simulink model "fftanalyzeri"  (R2012b)
settings: Solver=ode3  SolverMode=SingleTasking  StartTime=0.0  StopTime=20000  RelTol=1e-3
undefined symbols (not defined in the file or in its folder): pfb_coeff_gen_calc
undefined symbols (not defined in the file): fft_bin_flags_, magphmeanmem_, threshmem_
libraries: xbsIndex_r4 x9073, casper_library_misc x119, casper_library_flow_control x51, casper_library_delays x22, xps_library x10
(part 18 of 74)

== system fftanalyzeri/FIFO64_/FIFO32_0/FIFO16Cir_1/CounterArray2 ==
  chan : Inport
  inc : Inport  Port=2
  rst : Inport  Port=3
  chan2 : Inport  Port=4
  Mux : xbsIndex_r4/Mux  inputs=16  en=off  latency=0  precision=Full  arith_type=Unsigned  n_bits=16  bin_pt=14  quantization=Truncate  overflow=Wrap  dbl_ovrd=off  block_type=mux
  Mux1 : xbsIndex_r4/Mux  inputs=16  en=off  latency=0  precision=Full  arith_type=Unsigned  n_bits=16  bin_pt=14  quantization=Truncate  overflow=Wrap  dbl_ovrd=off  block_type=mux
  T1_4_{,1..15} (16 alike) : xbsIndex_r4/Counter  cnt_type=Free Running  cnt_to=Inf  operation=Up  start_count=0  cnt_by_val=1  arith_type=Unsigned  n_bits=8  bin_pt=0  load_pin=off  rst=on  en=on  explicit_period=on  period=1  dbl_ovrd=off  use_behavioral_HDL=off  implementation=Fabric  block_type=counter
  demux16_ : Subsystem
  Out1 : Outport
  Out2 : Outport  Port=2
  wires:
  chan/1 -> Mux/1, demux16_/1(Chan)
  inc/1 -> demux16_/2(din)
  rst/1 -> T1_4_9/1, T1_4_10/1, T1_4_11/1, T1_4_15/1, T1_4_8/1, T1_4_12/1, T1_4_14/1, T1_4_13/1, T1_4_7/1, T1_4_5/1, T1_4_1/1, T1_4_/1, T1_4_2/1, T1_4_3/1, T1_4_4/1, T1_4_6/1
  demux16_/1(Out1) -> T1_4_/2
  demux16_/2(Out2) -> T1_4_1/2
  demux16_/3(Out3) -> T1_4_2/2
  demux16_/4(Out4) -> T1_4_3/2
  demux16_/5(Out5) -> T1_4_4/2
  demux16_/6(Out6) -> T1_4_5/2
  demux16_/7(Out7) -> T1_4_6/2
  demux16_/8(Out8) -> T1_4_7/2
  demux16_/9(Out9) -> T1_4_9/2
  demux16_/10(Out10) -> T1_4_10/2
  demux16_/11(Out11) -> T1_4_11/2
  demux16_/12(Out12) -> T1_4_15/2
  demux16_/13(Out13) -> T1_4_8/2
  demux16_/14(Out14) -> T1_4_12/2
  demux16_/15(Out15) -> T1_4_13/2
  demux16_/16(Out16) -> T1_4_14/2
  T1_4_/1 -> Mux1/2, Mux/2
  T1_4_1/1 -> Mux1/3, Mux/3
  T1_4_2/1 -> Mux1/4, Mux/4
  T1_4_3/1 -> Mux1/5, Mux/5
  T1_4_4/1 -> Mux/6, Mux1/6
  T1_4_5/1 -> Mux1/7, Mux/7
  T1_4_6/1 -> Mux1/8, Mux/8
  T1_4_7/1 -> Mux1/9, Mux/9
  T1_4_9/1 -> Mux1/10, Mux/10
  T1_4_10/1 -> Mux1/11, Mux/11
  T1_4_11/1 -> Mux1/12, Mux/12
  T1_4_15/1 -> Mux1/13, Mux/13
  T1_4_8/1 -> Mux1/14, Mux/14
  T1_4_12/1 -> Mux1/15, Mux/15
  T1_4_13/1 -> Mux1/16, Mux/16
  T1_4_14/1 -> Mux/17, Mux1/17
  Mux/1 -> Out1/1
  chan2/1 -> Mux1/1
  Mux1/1 -> Out2/1

== system fftanalyzeri/FIFO64_/FIFO32_0/FIFO16Cir_2/CounterArray1 ==
  chan : Inport
  inc : Inport  Port=2
  rst : Inport  Port=3
  Mux : xbsIndex_r4/Mux  inputs=16  en=off  latency=0  precision=Full  arith_type=Unsigned  n_bits=16  bin_pt=14  quantization=Truncate  overflow=Wrap  dbl_ovrd=off  block_type=mux
  T1_4_{,1..15} (16 alike) : xbsIndex_r4/Counter  cnt_type=Free Running  cnt_to=Inf  operation=Up  start_count=0  cnt_by_val=1  arith_type=Unsigned  n_bits=8  bin_pt=0  load_pin=off  rst=on  en=on  explicit_period=on  period=1  dbl_ovrd=off  use_behavioral_HDL=off  implementation=Fabric  block_type=counter
  demux16_ : Subsystem
  Out1 : Outport
  wires:
  chan/1 -> Mux/1, demux16_/1(Chan)
  inc/1 -> demux16_/2(din)
  rst/1 -> T1_4_9/1, T1_4_10/1, T1_4_11/1, T1_4_12/1, T1_4_8/1, T1_4_13/1, T1_4_15/1, T1_4_14/1, T1_4_7/1, T1_4_6/1, T1_4_5/1, T1_4_4/1, T1_4_3/1, T1_4_2/1, T1_4_1/1, T1_4_/1
  demux16_/1(Out1) -> T1_4_/2
  demux16_/2(Out2) -> T1_4_1/2
  demux16_/3(Out3) -> T1_4_2/2
  demux16_/4(Out4) -> T1_4_3/2
  demux16_/5(Out5) -> T1_4_4/2
  demux16_/6(Out6) -> T1_4_5/2
  demux16_/7(Out7) -> T1_4_6/2
  demux16_/8(Out8) -> T1_4_7/2
  demux16_/9(Out9) -> T1_4_9/2
  demux16_/10(Out10) -> T1_4_10/2
  demux16_/11(Out11) -> T1_4_11/2
  demux16_/12(Out12) -> T1_4_12/2
  demux16_/13(Out13) -> T1_4_8/2
  demux16_/14(Out14) -> T1_4_13/2
  demux16_/15(Out15) -> T1_4_14/2
  demux16_/16(Out16) -> T1_4_15/2
  T1_4_/1 -> Mux/2
  T1_4_1/1 -> Mux/3
  T1_4_2/1 -> Mux/4
  T1_4_3/1 -> Mux/5
  T1_4_4/1 -> Mux/6
  T1_4_5/1 -> Mux/7
  T1_4_6/1 -> Mux/8
  T1_4_7/1 -> Mux/9
  T1_4_9/1 -> Mux/10
  T1_4_10/1 -> Mux/11
  T1_4_11/1 -> Mux/12
  T1_4_12/1 -> Mux/13
  T1_4_8/1 -> Mux/14
  T1_4_13/1 -> Mux/15
  T1_4_14/1 -> Mux/16
  T1_4_15/1 -> Mux/17
  Mux/1 -> Out1/1

== system fftanalyzeri/FIFO64_/FIFO32_0/FIFO16Cir_2/CounterArray2 ==
  chan : Inport
  inc : Inport  Port=2
  rst : Inport  Port=3
  chan2 : Inport  Port=4
  Mux : xbsIndex_r4/Mux  inputs=16  en=off  latency=0  precision=Full  arith_type=Unsigned  n_bits=16  bin_pt=14  quantization=Truncate  overflow=Wrap  dbl_ovrd=off  block_type=mux
  Mux1 : xbsIndex_r4/Mux  inputs=16  en=off  latency=0  precision=Full  arith_type=Unsigned  n_bits=16  bin_pt=14  quantization=Truncate  overflow=Wrap  dbl_ovrd=off  block_type=mux
  T1_4_{,1..15} (16 alike) : xbsIndex_r4/Counter  cnt_type=Free Running  cnt_to=Inf  operation=Up  start_count=0  cnt_by_val=1  arith_type=Unsigned  n_bits=8  bin_pt=0  load_pin=off  rst=on  en=on  explicit_period=on  period=1  dbl_ovrd=off  use_behavioral_HDL=off  implementation=Fabric  block_type=counter
  demux16_ : Subsystem
  Out1 : Outport
  Out2 : Outport  Port=2
  wires:
  chan/1 -> Mux/1, demux16_/1(Chan)
  inc/1 -> demux16_/2(din)
  rst/1 -> T1_4_9/1, T1_4_10/1, T1_4_11/1, T1_4_15/1, T1_4_8/1, T1_4_12/1, T1_4_14/1, T1_4_13/1, T1_4_7/1, T1_4_5/1, T1_4_1/1, T1_4_/1, T1_4_2/1, T1_4_3/1, T1_4_4/1, T1_4_6/1
  demux16_/1(Out1) -> T1_4_/2
  demux16_/2(Out2) -> T1_4_1/2
  demux16_/3(Out3) -> T1_4_2/2
  demux16_/4(Out4) -> T1_4_3/2
  demux16_/5(Out5) -> T1_4_4/2
  demux16_/6(Out6) -> T1_4_5/2
  demux16_/7(Out7) -> T1_4_6/2
  demux16_/8(Out8) -> T1_4_7/2
  demux16_/9(Out9) -> T1_4_9/2
  demux16_/10(Out10) -> T1_4_10/2
  demux16_/11(Out11) -> T1_4_11/2
  demux16_/12(Out12) -> T1_4_15/2
  demux16_/13(Out13) -> T1_4_8/2
  demux16_/14(Out14) -> T1_4_12/2
  demux16_/15(Out15) -> T1_4_13/2
  demux16_/16(Out16) -> T1_4_14/2
  T1_4_/1 -> Mux1/2, Mux/2
  T1_4_1/1 -> Mux1/3, Mux/3
  T1_4_2/1 -> Mux1/4, Mux/4
  T1_4_3/1 -> Mux1/5, Mux/5
  T1_4_4/1 -> Mux/6, Mux1/6
  T1_4_5/1 -> Mux1/7, Mux/7
  T1_4_6/1 -> Mux1/8, Mux/8
  T1_4_7/1 -> Mux1/9, Mux/9
  T1_4_9/1 -> Mux1/10, Mux/10
  T1_4_10/1 -> Mux1/11, Mux/11
  T1_4_11/1 -> Mux1/12, Mux/12
  T1_4_15/1 -> Mux1/13, Mux/13
  T1_4_8/1 -> Mux1/14, Mux/14
  T1_4_12/1 -> Mux1/15, Mux/15
  T1_4_13/1 -> Mux1/16, Mux/16
  T1_4_14/1 -> Mux/17, Mux1/17
  Mux/1 -> Out1/1
  chan2/1 -> Mux1/1
  Mux1/1 -> Out2/1

== system fftanalyzeri/FIFO64_/FIFO32_1/FIFO16Cir_1/CounterArray1 ==
  chan : Inport
  inc : Inport  Port=2
  rst : Inport  Port=3
  Mux : xbsIndex_r4/Mux  inputs=16  en=off  latency=0  precision=Full  arith_type=Unsigned  n_bits=16  bin_pt=14  quantization=Truncate  overflow=Wrap  dbl_ovrd=off  block_type=mux
  T1_4_{,1..15} (16 alike) : xbsIndex_r4/Counter  cnt_type=Free Running  cnt_to=Inf  operation=Up  start_count=0  cnt_by_val=1  arith_type=Unsigned  n_bits=8  bin_pt=0  load_pin=off  rst=on  en=on  explicit_period=on  period=1  dbl_ovrd=off  use_behavioral_HDL=off  implementation=Fabric  block_type=counter
  demux16_ : Subsystem
  Out1 : Outport
  wires:
  chan/1 -> Mux/1, demux16_/1(Chan)
  inc/1 -> demux16_/2(din)
  rst/1 -> T1_4_9/1, T1_4_10/1, T1_4_11/1, T1_4_12/1, T1_4_8/1, T1_4_13/1, T1_4_15/1, T1_4_14/1, T1_4_7/1, T1_4_6/1, T1_4_5/1, T1_4_4/1, T1_4_3/1, T1_4_2/1, T1_4_1/1, T1_4_/1
  demux16_/1(Out1) -> T1_4_/2
  demux16_/2(Out2) -> T1_4_1/2
  demux16_/3(Out3) -> T1_4_2/2
  demux16_/4(Out4) -> T1_4_3/2
  demux16_/5(Out5) -> T1_4_4/2
  demux16_/6(Out6) -> T1_4_5/2
  demux16_/7(Out7) -> T1_4_6/2
  demux16_/8(Out8) -> T1_4_7/2
  demux16_/9(Out9) -> T1_4_9/2
  demux16_/10(Out10) -> T1_4_10/2
  demux16_/11(Out11) -> T1_4_11/2
  demux16_/12(Out12) -> T1_4_12/2
  demux16_/13(Out13) -> T1_4_8/2
  demux16_/14(Out14) -> T1_4_13/2
  demux16_/15(Out15) -> T1_4_14/2
  demux16_/16(Out16) -> T1_4_15/2
  T1_4_/1 -> Mux/2
  T1_4_1/1 -> Mux/3
  T1_4_2/1 -> Mux/4
  T1_4_3/1 -> Mux/5
  T1_4_4/1 -> Mux/6
  T1_4_5/1 -> Mux/7
  T1_4_6/1 -> Mux/8
  T1_4_7/1 -> Mux/9
  T1_4_9/1 -> Mux/10
  T1_4_10/1 -> Mux/11
  T1_4_11/1 -> Mux/12
  T1_4_12/1 -> Mux/13
  T1_4_8/1 -> Mux/14
  T1_4_13/1 -> Mux/15
  T1_4_14/1 -> Mux/16
  T1_4_15/1 -> Mux/17
  Mux/1 -> Out1/1

== system fftanalyzeri/FIFO64_/FIFO32_1/FIFO16Cir_1/CounterArray2 ==
  chan : Inport
  inc : Inport  Port=2
  rst : Inport  Port=3
  chan2 : Inport  Port=4
  Mux : xbsIndex_r4/Mux  inputs=16  en=off  latency=0  precision=Full  arith_type=Unsigned  n_bits=16  bin_pt=14  quantization=Truncate  overflow=Wrap  dbl_ovrd=off  block_type=mux
  Mux1 : xbsIndex_r4/Mux  inputs=16  en=off  latency=0  precision=Full  arith_type=Unsigned  n_bits=16  bin_pt=14  quantization=Truncate  overflow=Wrap  dbl_ovrd=off  block_type=mux
  T1_4_{,1..15} (16 alike) : xbsIndex_r4/Counter  cnt_type=Free Running  cnt_to=Inf  operation=Up  start_count=0  cnt_by_val=1  arith_type=Unsigned  n_bits=8  bin_pt=0  load_pin=off  rst=on  en=on  explicit_period=on  period=1  dbl_ovrd=off  use_behavioral_HDL=off  implementation=Fabric  block_type=counter
  demux16_ : Subsystem
  Out1 : Outport
  Out2 : Outport  Port=2
  wires:
  chan/1 -> Mux/1, demux16_/1(Chan)
  inc/1 -> demux16_/2(din)
  rst/1 -> T1_4_9/1, T1_4_10/1, T1_4_11/1, T1_4_15/1, T1_4_8/1, T1_4_12/1, T1_4_14/1, T1_4_13/1, T1_4_7/1, T1_4_5/1, T1_4_1/1, T1_4_/1, T1_4_2/1, T1_4_3/1, T1_4_4/1, T1_4_6/1
  demux16_/1(Out1) -> T1_4_/2
  demux16_/2(Out2) -> T1_4_1/2
  demux16_/3(Out3) -> T1_4_2/2
  demux16_/4(Out4) -> T1_4_3/2
  demux16_/5(Out5) -> T1_4_4/2
  demux16_/6(Out6) -> T1_4_5/2
  demux16_/7(Out7) -> T1_4_6/2
  demux16_/8(Out8) -> T1_4_7/2
  demux16_/9(Out9) -> T1_4_9/2
  demux16_/10(Out10) -> T1_4_10/2
  demux16_/11(Out11) -> T1_4_11/2
  demux16_/12(Out12) -> T1_4_15/2
  demux16_/13(Out13) -> T1_4_8/2
  demux16_/14(Out14) -> T1_4_12/2
  demux16_/15(Out15) -> T1_4_13/2
  demux16_/16(Out16) -> T1_4_14/2
  T1_4_/1 -> Mux1/2, Mux/2
  T1_4_1/1 -> Mux1/3, Mux/3
  T1_4_2/1 -> Mux1/4, Mux/4
  T1_4_3/1 -> Mux1/5, Mux/5
  T1_4_4/1 -> Mux/6, Mux1/6
  T1_4_5/1 -> Mux1/7, Mux/7
  T1_4_6/1 -> Mux1/8, Mux/8
  T1_4_7/1 -> Mux1/9, Mux/9
  T1_4_9/1 -> Mux1/10, Mux/10
  T1_4_10/1 -> Mux1/11, Mux/11
  T1_4_11/1 -> Mux1/12, Mux/12
  T1_4_15/1 -> Mux1/13, Mux/13
  T1_4_8/1 -> Mux1/14, Mux/14
  T1_4_12/1 -> Mux1/15, Mux/15
  T1_4_13/1 -> Mux1/16, Mux/16
  T1_4_14/1 -> Mux/17, Mux1/17
  Mux/1 -> Out1/1
  chan2/1 -> Mux1/1
  Mux1/1 -> Out2/1

== system fftanalyzeri/FIFO64_/FIFO32_1/FIFO16Cir_2/CounterArray1 ==
  chan : Inport
  inc : Inport  Port=2
  rst : Inport  Port=3
  Mux : xbsIndex_r4/Mux  inputs=16  en=off  latency=0  precision=Full  arith_type=Unsigned  n_bits=16  bin_pt=14  quantization=Truncate  overflow=Wrap  dbl_ovrd=off  block_type=mux
  T1_4_{,1..15} (16 alike) : xbsIndex_r4/Counter  cnt_type=Free Running  cnt_to=Inf  operation=Up  start_count=0  cnt_by_val=1  arith_type=Unsigned  n_bits=8  bin_pt=0  load_pin=off  rst=on  en=on  explicit_period=on  period=1  dbl_ovrd=off  use_behavioral_HDL=off  implementation=Fabric  block_type=counter
  demux16_ : Subsystem
  Out1 : Outport
  wires:
  chan/1 -> Mux/1, demux16_/1(Chan)
  inc/1 -> demux16_/2(din)
  rst/1 -> T1_4_9/1, T1_4_10/1, T1_4_11/1, T1_4_12/1, T1_4_8/1, T1_4_13/1, T1_4_15/1, T1_4_14/1, T1_4_7/1, T1_4_6/1, T1_4_5/1, T1_4_4/1, T1_4_3/1, T1_4_2/1, T1_4_1/1, T1_4_/1
  demux16_/1(Out1) -> T1_4_/2
  demux16_/2(Out2) -> T1_4_1/2
  demux16_/3(Out3) -> T1_4_2/2
  demux16_/4(Out4) -> T1_4_3/2
  demux16_/5(Out5) -> T1_4_4/2
  demux16_/6(Out6) -> T1_4_5/2
  demux16_/7(Out7) -> T1_4_6/2
  demux16_/8(Out8) -> T1_4_7/2
  demux16_/9(Out9) -> T1_4_9/2
  demux16_/10(Out10) -> T1_4_10/2
  demux16_/11(Out11) -> T1_4_11/2
  demux16_/12(Out12) -> T1_4_12/2
  demux16_/13(Out13) -> T1_4_8/2
  demux16_/14(Out14) -> T1_4_13/2
  demux16_/15(Out15) -> T1_4_14/2
  demux16_/16(Out16) -> T1_4_15/2
  T1_4_/1 -> Mux/2
  T1_4_1/1 -> Mux/3
  T1_4_2/1 -> Mux/4
  T1_4_3/1 -> Mux/5
  T1_4_4/1 -> Mux/6
  T1_4_5/1 -> Mux/7
  T1_4_6/1 -> Mux/8
  T1_4_7/1 -> Mux/9
  T1_4_9/1 -> Mux/10
  T1_4_10/1 -> Mux/11
  T1_4_11/1 -> Mux/12
  T1_4_12/1 -> Mux/13
  T1_4_8/1 -> Mux/14
  T1_4_13/1 -> Mux/15
  T1_4_14/1 -> Mux/16
  T1_4_15/1 -> Mux/17
  Mux/1 -> Out1/1

== system fftanalyzeri/FIFO64_/FIFO32_1/FIFO16Cir_2/CounterArray2 ==
  chan : Inport
  inc : Inport  Port=2
  rst : Inport  Port=3
  chan2 : Inport  Port=4
  Mux : xbsIndex_r4/Mux  inputs=16  en=off  latency=0  precision=Full  arith_type=Unsigned  n_bits=16  bin_pt=14  quantization=Truncate  overflow=Wrap  dbl_ovrd=off  block_type=mux
  Mux1 : xbsIndex_r4/Mux  inputs=16  en=off  latency=0  precision=Full  arith_type=Unsigned  n_bits=16  bin_pt=14  quantization=Truncate  overflow=Wrap  dbl_ovrd=off  block_type=mux
  T1_4_{,1..15} (16 alike) : xbsIndex_r4/Counter  cnt_type=Free Running  cnt_to=Inf  operation=Up  start_count=0  cnt_by_val=1  arith_type=Unsigned  n_bits=8  bin_pt=0  load_pin=off  rst=on  en=on  explicit_period=on  period=1  dbl_ovrd=off  use_behavioral_HDL=off  implementation=Fabric  block_type=counter
  demux16_ : Subsystem
  Out1 : Outport
  Out2 : Outport  Port=2
  wires:
  chan/1 -> Mux/1, demux16_/1(Chan)
  inc/1 -> demux16_/2(din)
  rst/1 -> T1_4_9/1, T1_4_10/1, T1_4_11/1, T1_4_15/1, T1_4_8/1, T1_4_12/1, T1_4_14/1, T1_4_13/1, T1_4_7/1, T1_4_5/1, T1_4_1/1, T1_4_/1, T1_4_2/1, T1_4_3/1, T1_4_4/1, T1_4_6/1
  demux16_/1(Out1) -> T1_4_/2
  demux16_/2(Out2) -> T1_4_1/2
  demux16_/3(Out3) -> T1_4_2/2
  demux16_/4(Out4) -> T1_4_3/2
  demux16_/5(Out5) -> T1_4_4/2
  demux16_/6(Out6) -> T1_4_5/2
  demux16_/7(Out7) -> T1_4_6/2
  demux16_/8(Out8) -> T1_4_7/2
  demux16_/9(Out9) -> T1_4_9/2
  demux16_/10(Out10) -> T1_4_10/2
  demux16_/11(Out11) -> T1_4_11/2
  demux16_/12(Out12) -> T1_4_15/2
  demux16_/13(Out13) -> T1_4_8/2
  demux16_/14(Out14) -> T1_4_12/2
  demux16_/15(Out15) -> T1_4_13/2
  demux16_/16(Out16) -> T1_4_14/2
  T1_4_/1 -> Mux1/2, Mux/2
  T1_4_1/1 -> Mux1/3, Mux/3
  T1_4_2/1 -> Mux1/4, Mux/4
  T1_4_3/1 -> Mux1/5, Mux/5
  T1_4_4/1 -> Mux/6, Mux1/6
  T1_4_5/1 -> Mux1/7, Mux/7
  T1_4_6/1 -> Mux1/8, Mux/8
  T1_4_7/1 -> Mux1/9, Mux/9
  T1_4_9/1 -> Mux1/10, Mux/10
  T1_4_10/1 -> Mux1/11, Mux/11
  T1_4_11/1 -> Mux1/12, Mux/12
  T1_4_15/1 -> Mux1/13, Mux/13
  T1_4_8/1 -> Mux1/14, Mux/14
  T1_4_12/1 -> Mux1/15, Mux/15
  T1_4_13/1 -> Mux1/16, Mux/16
  T1_4_14/1 -> Mux/17, Mux1/17
  Mux/1 -> Out1/1
  chan2/1 -> Mux1/1
  Mux1/1 -> Out2/1

== system fftanalyzeri/FIFO64_1/FIFO32_0/FIFO16Cir_1/CounterArray1 ==
  chan : Inport
  inc : Inport  Port=2
  rst : Inport  Port=3
  Mux : xbsIndex_r4/Mux  inputs=16  en=off  latency=0  precision=Full  arith_type=Unsigned  n_bits=16  bin_pt=14  quantization=Truncate  overflow=Wrap  dbl_ovrd=off  block_type=mux
  T1_4_{,1..15} (16 alike) : xbsIndex_r4/Counter  cnt_type=Free Running  cnt_to=Inf  operation=Up  start_count=0  cnt_by_val=1  arith_type=Unsigned  n_bits=8  bin_pt=0  load_pin=off  rst=on  en=on  explicit_period=on  period=1  dbl_ovrd=off  use_behavioral_HDL=off  implementation=Fabric  block_type=counter
  demux16_ : Subsystem
  Out1 : Outport
  wires:
  chan/1 -> Mux/1, demux16_/1(Chan)
  inc/1 -> demux16_/2(din)
  rst/1 -> T1_4_9/1, T1_4_10/1, T1_4_11/1, T1_4_12/1, T1_4_8/1, T1_4_13/1, T1_4_15/1, T1_4_14/1, T1_4_7/1, T1_4_6/1, T1_4_5/1, T1_4_4/1, T1_4_3/1, T1_4_2/1, T1_4_1/1, T1_4_/1
  demux16_/1(Out1) -> T1_4_/2
  demux16_/2(Out2) -> T1_4_1/2
  demux16_/3(Out3) -> T1_4_2/2
  demux16_/4(Out4) -> T1_4_3/2
  demux16_/5(Out5) -> T1_4_4/2
  demux16_/6(Out6) -> T1_4_5/2
  demux16_/7(Out7) -> T1_4_6/2
  demux16_/8(Out8) -> T1_4_7/2
  demux16_/9(Out9) -> T1_4_9/2
  demux16_/10(Out10) -> T1_4_10/2
  demux16_/11(Out11) -> T1_4_11/2
  demux16_/12(Out12) -> T1_4_12/2
  demux16_/13(Out13) -> T1_4_8/2
  demux16_/14(Out14) -> T1_4_13/2
  demux16_/15(Out15) -> T1_4_14/2
  demux16_/16(Out16) -> T1_4_15/2
  T1_4_/1 -> Mux/2
  T1_4_1/1 -> Mux/3
  T1_4_2/1 -> Mux/4
  T1_4_3/1 -> Mux/5
  T1_4_4/1 -> Mux/6
  T1_4_5/1 -> Mux/7
  T1_4_6/1 -> Mux/8
  T1_4_7/1 -> Mux/9
  T1_4_9/1 -> Mux/10
  T1_4_10/1 -> Mux/11
  T1_4_11/1 -> Mux/12
  T1_4_12/1 -> Mux/13
  T1_4_8/1 -> Mux/14
  T1_4_13/1 -> Mux/15
  T1_4_14/1 -> Mux/16
  T1_4_15/1 -> Mux/17
  Mux/1 -> Out1/1

== system fftanalyzeri/FIFO64_1/FIFO32_0/FIFO16Cir_1/CounterArray2 ==
  chan : Inport
  inc : Inport  Port=2
  rst : Inport  Port=3
  chan2 : Inport  Port=4
  Mux : xbsIndex_r4/Mux  inputs=16  en=off  latency=0  precision=Full  arith_type=Unsigned  n_bits=16  bin_pt=14  quantization=Truncate  overflow=Wrap  dbl_ovrd=off  block_type=mux
  Mux1 : xbsIndex_r4/Mux  inputs=16  en=off  latency=0  precision=Full  arith_type=Unsigned  n_bits=16  bin_pt=14  quantization=Truncate  overflow=Wrap  dbl_ovrd=off  block_type=mux
  T1_4_{,1..15} (16 alike) : xbsIndex_r4/Counter  cnt_type=Free Running  cnt_to=Inf  operation=Up  start_count=0  cnt_by_val=1  arith_type=Unsigned  n_bits=8  bin_pt=0  load_pin=off  rst=on  en=on  explicit_period=on  period=1  dbl_ovrd=off  use_behavioral_HDL=off  implementation=Fabric  block_type=counter
  demux16_ : Subsystem
  Out1 : Outport
  Out2 : Outport  Port=2
  wires:
  chan/1 -> Mux/1, demux16_/1(Chan)
  inc/1 -> demux16_/2(din)
  rst/1 -> T1_4_9/1, T1_4_10/1, T1_4_11/1, T1_4_15/1, T1_4_8/1, T1_4_12/1, T1_4_14/1, T1_4_13/1, T1_4_7/1, T1_4_5/1, T1_4_1/1, T1_4_/1, T1_4_2/1, T1_4_3/1, T1_4_4/1, T1_4_6/1
  demux16_/1(Out1) -> T1_4_/2
  demux16_/2(Out2) -> T1_4_1/2
  demux16_/3(Out3) -> T1_4_2/2
  demux16_/4(Out4) -> T1_4_3/2
  demux16_/5(Out5) -> T1_4_4/2
  demux16_/6(Out6) -> T1_4_5/2
  demux16_/7(Out7) -> T1_4_6/2
  demux16_/8(Out8) -> T1_4_7/2
  demux16_/9(Out9) -> T1_4_9/2
  demux16_/10(Out10) -> T1_4_10/2
  demux16_/11(Out11) -> T1_4_11/2
  demux16_/12(Out12) -> T1_4_15/2
  demux16_/13(Out13) -> T1_4_8/2
  demux16_/14(Out14) -> T1_4_12/2
  demux16_/15(Out15) -> T1_4_13/2
  demux16_/16(Out16) -> T1_4_14/2
  T1_4_/1 -> Mux1/2, Mux/2
  T1_4_1/1 -> Mux1/3, Mux/3
  T1_4_2/1 -> Mux1/4, Mux/4
  T1_4_3/1 -> Mux1/5, Mux/5
  T1_4_4/1 -> Mux/6, Mux1/6
  T1_4_5/1 -> Mux1/7, Mux/7
  T1_4_6/1 -> Mux1/8, Mux/8
  T1_4_7/1 -> Mux1/9, Mux/9
  T1_4_9/1 -> Mux1/10, Mux/10
  T1_4_10/1 -> Mux1/11, Mux/11
  T1_4_11/1 -> Mux1/12, Mux/12
  T1_4_15/1 -> Mux1/13, Mux/13
  T1_4_8/1 -> Mux1/14, Mux/14
  T1_4_12/1 -> Mux1/15, Mux/15
  T1_4_13/1 -> Mux1/16, Mux/16
  T1_4_14/1 -> Mux/17, Mux1/17
  Mux/1 -> Out1/1
  chan2/1 -> Mux1/1
  Mux1/1 -> Out2/1

== system fftanalyzeri/FIFO64_1/FIFO32_0/FIFO16Cir_2/CounterArray1 ==
  chan : Inport
  inc : Inport  Port=2
  rst : Inport  Port=3
  Mux : xbsIndex_r4/Mux  inputs=16  en=off  latency=0  precision=Full  arith_type=Unsigned  n_bits=16  bin_pt=14  quantization=Truncate  overflow=Wrap  dbl_ovrd=off  block_type=mux
  T1_4_{,1..15} (16 alike) : xbsIndex_r4/Counter  cnt_type=Free Running  cnt_to=Inf  operation=Up  start_count=0  cnt_by_val=1  arith_type=Unsigned  n_bits=8  bin_pt=0  load_pin=off  rst=on  en=on  explicit_period=on  period=1  dbl_ovrd=off  use_behavioral_HDL=off  implementation=Fabric  block_type=counter
  demux16_ : Subsystem
  Out1 : Outport
  wires:
  chan/1 -> Mux/1, demux16_/1(Chan)
  inc/1 -> demux16_/2(din)
  rst/1 -> T1_4_9/1, T1_4_10/1, T1_4_11/1, T1_4_12/1, T1_4_8/1, T1_4_13/1, T1_4_15/1, T1_4_14/1, T1_4_7/1, T1_4_6/1, T1_4_5/1, T1_4_4/1, T1_4_3/1, T1_4_2/1, T1_4_1/1, T1_4_/1
  demux16_/1(Out1) -> T1_4_/2
  demux16_/2(Out2) -> T1_4_1/2
  demux16_/3(Out3) -> T1_4_2/2
  demux16_/4(Out4) -> T1_4_3/2
  demux16_/5(Out5) -> T1_4_4/2
  demux16_/6(Out6) -> T1_4_5/2
  demux16_/7(Out7) -> T1_4_6/2
  demux16_/8(Out8) -> T1_4_7/2
  demux16_/9(Out9) -> T1_4_9/2
  demux16_/10(Out10) -> T1_4_10/2
  demux16_/11(Out11) -> T1_4_11/2
  demux16_/12(Out12) -> T1_4_12/2
  demux16_/13(Out13) -> T1_4_8/2
  demux16_/14(Out14) -> T1_4_13/2
  demux16_/15(Out15) -> T1_4_14/2
  demux16_/16(Out16) -> T1_4_15/2
  T1_4_/1 -> Mux/2
  T1_4_1/1 -> Mux/3
  T1_4_2/1 -> Mux/4
  T1_4_3/1 -> Mux/5
  T1_4_4/1 -> Mux/6
  T1_4_5/1 -> Mux/7
  T1_4_6/1 -> Mux/8
  T1_4_7/1 -> Mux/9
  T1_4_9/1 -> Mux/10
  T1_4_10/1 -> Mux/11
  T1_4_11/1 -> Mux/12
  T1_4_12/1 -> Mux/13
  T1_4_8/1 -> Mux/14
  T1_4_13/1 -> Mux/15
  T1_4_14/1 -> Mux/16
  T1_4_15/1 -> Mux/17
  Mux/1 -> Out1/1

== system fftanalyzeri/FIFO64_1/FIFO32_0/FIFO16Cir_2/CounterArray2 ==
  chan : Inport
  inc : Inport  Port=2
  rst : Inport  Port=3
  chan2 : Inport  Port=4
  Mux : xbsIndex_r4/Mux  inputs=16  en=off  latency=0  precision=Full  arith_type=Unsigned  n_bits=16  bin_pt=14  quantization=Truncate  overflow=Wrap  dbl_ovrd=off  block_type=mux
  Mux1 : xbsIndex_r4/Mux  inputs=16  en=off  latency=0  precision=Full  arith_type=Unsigned  n_bits=16  bin_pt=14  quantization=Truncate  overflow=Wrap  dbl_ovrd=off  block_type=mux
  T1_4_{,1..15} (16 alike) : xbsIndex_r4/Counter  cnt_type=Free Running  cnt_to=Inf  operation=Up  start_count=0  cnt_by_val=1  arith_type=Unsigned  n_bits=8  bin_pt=0  load_pin=off  rst=on  en=on  explicit_period=on  period=1  dbl_ovrd=off  use_behavioral_HDL=off  implementation=Fabric  block_type=counter
  demux16_ : Subsystem
  Out1 : Outport
  Out2 : Outport  Port=2
  wires:
  chan/1 -> Mux/1, demux16_/1(Chan)
  inc/1 -> demux16_/2(din)
  rst/1 -> T1_4_9/1, T1_4_10/1, T1_4_11/1, T1_4_15/1, T1_4_8/1, T1_4_12/1, T1_4_14/1, T1_4_13/1, T1_4_7/1, T1_4_5/1, T1_4_1/1, T1_4_/1, T1_4_2/1, T1_4_3/1, T1_4_4/1, T1_4_6/1
  demux16_/1(Out1) -> T1_4_/2
  demux16_/2(Out2) -> T1_4_1/2
  demux16_/3(Out3) -> T1_4_2/2
  demux16_/4(Out4) -> T1_4_3/2
  demux16_/5(Out5) -> T1_4_4/2
  demux16_/6(Out6) -> T1_4_5/2
  demux16_/7(Out7) -> T1_4_6/2
  demux16_/8(Out8) -> T1_4_7/2
  demux16_/9(Out9) -> T1_4_9/2
  demux16_/10(Out10) -> T1_4_10/2
  demux16_/11(Out11) -> T1_4_11/2
  demux16_/12(Out12) -> T1_4_15/2
  demux16_/13(Out13) -> T1_4_8/2
  demux16_/14(Out14) -> T1_4_12/2
  demux16_/15(Out15) -> T1_4_13/2
  demux16_/16(Out16) -> T1_4_14/2
  T1_4_/1 -> Mux1/2, Mux/2
  T1_4_1/1 -> Mux1/3, Mux/3
  T1_4_2/1 -> Mux1/4, Mux/4
  T1_4_3/1 -> Mux1/5, Mux/5
  T1_4_4/1 -> Mux/6, Mux1/6
  T1_4_5/1 -> Mux1/7, Mux/7
  T1_4_6/1 -> Mux1/8, Mux/8
  T1_4_7/1 -> Mux1/9, Mux/9
  T1_4_9/1 -> Mux1/10, Mux/10
  T1_4_10/1 -> Mux1/11, Mux/11
  T1_4_11/1 -> Mux1/12, Mux/12
  T1_4_15/1 -> Mux1/13, Mux/13
  T1_4_8/1 -> Mux1/14, Mux/14
  T1_4_12/1 -> Mux1/15, Mux/15
  T1_4_13/1 -> Mux1/16, Mux/16
  T1_4_14/1 -> Mux/17, Mux1/17
  Mux/1 -> Out1/1
  chan2/1 -> Mux1/1
  Mux1/1 -> Out2/1

== system fftanalyzeri/FIFO64_1/FIFO32_1/FIFO16Cir_1/CounterArray1 ==
  chan : Inport
  inc : Inport  Port=2
  rst : Inport  Port=3
  Mux : xbsIndex_r4/Mux  inputs=16  en=off  latency=0  precision=Full  arith_type=Unsigned  n_bits=16  bin_pt=14  quantization=Truncate  overflow=Wrap  dbl_ovrd=off  block_type=mux
  T1_4_{,1..15} (16 alike) : xbsIndex_r4/Counter  cnt_type=Free Running  cnt_to=Inf  operation=Up  start_count=0  cnt_by_val=1  arith_type=Unsigned  n_bits=8  bin_pt=0  load_pin=off  rst=on  en=on  explicit_period=on  period=1  dbl_ovrd=off  use_behavioral_HDL=off  implementation=Fabric  block_type=counter
  demux16_ : Subsystem
  Out1 : Outport
  wires:
  chan/1 -> Mux/1, demux16_/1(Chan)
  inc/1 -> demux16_/2(din)
  rst/1 -> T1_4_9/1, T1_4_10/1, T1_4_11/1, T1_4_12/1, T1_4_8/1, T1_4_13/1, T1_4_15/1, T1_4_14/1, T1_4_7/1, T1_4_6/1, T1_4_5/1, T1_4_4/1, T1_4_3/1, T1_4_2/1, T1_4_1/1, T1_4_/1
  demux16_/1(Out1) -> T1_4_/2
  demux16_/2(Out2) -> T1_4_1/2
  demux16_/3(Out3) -> T1_4_2/2
  demux16_/4(Out4) -> T1_4_3/2
  demux16_/5(Out5) -> T1_4_4/2
  demux16_/6(Out6) -> T1_4_5/2
  demux16_/7(Out7) -> T1_4_6/2
  demux16_/8(Out8) -> T1_4_7/2
  demux16_/9(Out9) -> T1_4_9/2
  demux16_/10(Out10) -> T1_4_10/2
  demux16_/11(Out11) -> T1_4_11/2
  demux16_/12(Out12) -> T1_4_12/2
  demux16_/13(Out13) -> T1_4_8/2
  demux16_/14(Out14) -> T1_4_13/2
  demux16_/15(Out15) -> T1_4_14/2
  demux16_/16(Out16) -> T1_4_15/2
  T1_4_/1 -> Mux/2
  T1_4_1/1 -> Mux/3
  T1_4_2/1 -> Mux/4
  T1_4_3/1 -> Mux/5
  T1_4_4/1 -> Mux/6
  T1_4_5/1 -> Mux/7
  T1_4_6/1 -> Mux/8
  T1_4_7/1 -> Mux/9
  T1_4_9/1 -> Mux/10
  T1_4_10/1 -> Mux/11
  T1_4_11/1 -> Mux/12
  T1_4_12/1 -> Mux/13
  T1_4_8/1 -> Mux/14
  T1_4_13/1 -> Mux/15
  T1_4_14/1 -> Mux/16
  T1_4_15/1 -> Mux/17
  Mux/1 -> Out1/1

== system fftanalyzeri/FIFO64_1/FIFO32_1/FIFO16Cir_1/CounterArray2 ==
  chan : Inport
  inc : Inport  Port=2
  rst : Inport  Port=3
  chan2 : Inport  Port=4
  Mux : xbsIndex_r4/Mux  inputs=16  en=off  latency=0  precision=Full  arith_type=Unsigned  n_bits=16  bin_pt=14  quantization=Truncate  overflow=Wrap  dbl_ovrd=off  block_type=mux
  Mux1 : xbsIndex_r4/Mux  inputs=16  en=off  latency=0  precision=Full  arith_type=Unsigned  n_bits=16  bin_pt=14  quantization=Truncate  overflow=Wrap  dbl_ovrd=off  block_type=mux
  T1_4_{,1..15} (16 alike) : xbsIndex_r4/Counter  cnt_type=Free Running  cnt_to=Inf  operation=Up  start_count=0  cnt_by_val=1  arith_type=Unsigned  n_bits=8  bin_pt=0  load_pin=off  rst=on  en=on  explicit_period=on  period=1  dbl_ovrd=off  use_behavioral_HDL=off  implementation=Fabric  block_type=counter
  demux16_ : Subsystem
  Out1 : Outport
  Out2 : Outport  Port=2
  wires:
  chan/1 -> Mux/1, demux16_/1(Chan)
  inc/1 -> demux16_/2(din)
  rst/1 -> T1_4_9/1, T1_4_10/1, T1_4_11/1, T1_4_15/1, T1_4_8/1, T1_4_12/1, T1_4_14/1, T1_4_13/1, T1_4_7/1, T1_4_5/1, T1_4_1/1, T1_4_/1, T1_4_2/1, T1_4_3/1, T1_4_4/1, T1_4_6/1
  demux16_/1(Out1) -> T1_4_/2
  demux16_/2(Out2) -> T1_4_1/2
  demux16_/3(Out3) -> T1_4_2/2
  demux16_/4(Out4) -> T1_4_3/2
  demux16_/5(Out5) -> T1_4_4/2
  demux16_/6(Out6) -> T1_4_5/2
  demux16_/7(Out7) -> T1_4_6/2
  demux16_/8(Out8) -> T1_4_7/2
  demux16_/9(Out9) -> T1_4_9/2
  demux16_/10(Out10) -> T1_4_10/2
  demux16_/11(Out11) -> T1_4_11/2
  demux16_/12(Out12) -> T1_4_15/2
  demux16_/13(Out13) -> T1_4_8/2
  demux16_/14(Out14) -> T1_4_12/2
  demux16_/15(Out15) -> T1_4_13/2
  demux16_/16(Out16) -> T1_4_14/2
  T1_4_/1 -> Mux1/2, Mux/2
  T1_4_1/1 -> Mux1/3, Mux/3
  T1_4_2/1 -> Mux1/4, Mux/4
  T1_4_3/1 -> Mux1/5, Mux/5
  T1_4_4/1 -> Mux/6, Mux1/6
  T1_4_5/1 -> Mux1/7, Mux/7
  T1_4_6/1 -> Mux1/8, Mux/8
  T1_4_7/1 -> Mux1/9, Mux/9
  T1_4_9/1 -> Mux1/10, Mux/10
  T1_4_10/1 -> Mux1/11, Mux/11
  T1_4_11/1 -> Mux1/12, Mux/12
  T1_4_15/1 -> Mux1/13, Mux/13
  T1_4_8/1 -> Mux1/14, Mux/14
  T1_4_12/1 -> Mux1/15, Mux/15
  T1_4_13/1 -> Mux1/16, Mux/16
  T1_4_14/1 -> Mux/17, Mux1/17
  Mux/1 -> Out1/1
  chan2/1 -> Mux1/1
  Mux1/1 -> Out2/1

== system fftanalyzeri/FIFO64_1/FIFO32_1/FIFO16Cir_2/CounterArray1 ==
  chan : Inport
  inc : Inport  Port=2
  rst : Inport  Port=3
  Mux : xbsIndex_r4/Mux  inputs=16  en=off  latency=0  precision=Full  arith_type=Unsigned  n_bits=16  bin_pt=14  quantization=Truncate  overflow=Wrap  dbl_ovrd=off  block_type=mux
  T1_4_{,1..15} (16 alike) : xbsIndex_r4/Counter  cnt_type=Free Running  cnt_to=Inf  operation=Up  start_count=0  cnt_by_val=1  arith_type=Unsigned  n_bits=8  bin_pt=0  load_pin=off  rst=on  en=on  explicit_period=on  period=1  dbl_ovrd=off  use_behavioral_HDL=off  implementation=Fabric  block_type=counter
  demux16_ : Subsystem
  Out1 : Outport
  wires:
  chan/1 -> Mux/1, demux16_/1(Chan)
  inc/1 -> demux16_/2(din)
  rst/1 -> T1_4_9/1, T1_4_10/1, T1_4_11/1, T1_4_12/1, T1_4_8/1, T1_4_13/1, T1_4_15/1, T1_4_14/1, T1_4_7/1, T1_4_6/1, T1_4_5/1, T1_4_4/1, T1_4_3/1, T1_4_2/1, T1_4_1/1, T1_4_/1
  demux16_/1(Out1) -> T1_4_/2
  demux16_/2(Out2) -> T1_4_1/2
  demux16_/3(Out3) -> T1_4_2/2
  demux16_/4(Out4) -> T1_4_3/2
  demux16_/5(Out5) -> T1_4_4/2
  demux16_/6(Out6) -> T1_4_5/2
  demux16_/7(Out7) -> T1_4_6/2
  demux16_/8(Out8) -> T1_4_7/2
  demux16_/9(Out9) -> T1_4_9/2
  demux16_/10(Out10) -> T1_4_10/2
  demux16_/11(Out11) -> T1_4_11/2
  demux16_/12(Out12) -> T1_4_12/2
  demux16_/13(Out13) -> T1_4_8/2
  demux16_/14(Out14) -> T1_4_13/2
  demux16_/15(Out15) -> T1_4_14/2
  demux16_/16(Out16) -> T1_4_15/2
  T1_4_/1 -> Mux/2
  T1_4_1/1 -> Mux/3
  T1_4_2/1 -> Mux/4
  T1_4_3/1 -> Mux/5
  T1_4_4/1 -> Mux/6
  T1_4_5/1 -> Mux/7
  T1_4_6/1 -> Mux/8
  T1_4_7/1 -> Mux/9
  T1_4_9/1 -> Mux/10
  T1_4_10/1 -> Mux/11
  T1_4_11/1 -> Mux/12
  T1_4_12/1 -> Mux/13
  T1_4_8/1 -> Mux/14
  T1_4_13/1 -> Mux/15
  T1_4_14/1 -> Mux/16
  T1_4_15/1 -> Mux/17
  Mux/1 -> Out1/1

== system fftanalyzeri/FIFO64_1/FIFO32_1/FIFO16Cir_2/CounterArray2 ==
  chan : Inport
  inc : Inport  Port=2
  rst : Inport  Port=3
  chan2 : Inport  Port=4
  Mux : xbsIndex_r4/Mux  inputs=16  en=off  latency=0  precision=Full  arith_type=Unsigned  n_bits=16  bin_pt=14  quantization=Truncate  overflow=Wrap  dbl_ovrd=off  block_type=mux
  Mux1 : xbsIndex_r4/Mux  inputs=16  en=off  latency=0  precision=Full  arith_type=Unsigned  n_bits=16  bin_pt=14  quantization=Truncate  overflow=Wrap  dbl_ovrd=off  block_type=mux
  T1_4_{,1..15} (16 alike) : xbsIndex_r4/Counter  cnt_type=Free Running  cnt_to=Inf  operation=Up  start_count=0  cnt_by_val=1  arith_type=Unsigned  n_bits=8  bin_pt=0  load_pin=off  rst=on  en=on  explicit_period=on  period=1  dbl_ovrd=off  use_behavioral_HDL=off  implementation=Fabric  block_type=counter
  demux16_ : Subsystem
  Out1 : Outport
  Out2 : Outport  Port=2
  wires:
  chan/1 -> Mux/1, demux16_/1(Chan)
  inc/1 -> demux16_/2(din)
  rst/1 -> T1_4_9/1, T1_4_10/1, T1_4_11/1, T1_4_15/1, T1_4_8/1, T1_4_12/1, T1_4_14/1, T1_4_13/1, T1_4_7/1, T1_4_5/1, T1_4_1/1, T1_4_/1, T1_4_2/1, T1_4_3/1, T1_4_4/1, T1_4_6/1
  demux16_/1(Out1) -> T1_4_/2
  demux16_/2(Out2) -> T1_4_1/2
  demux16_/3(Out3) -> T1_4_2/2
  demux16_/4(Out4) -> T1_4_3/2
  demux16_/5(Out5) -> T1_4_4/2
  demux16_/6(Out6) -> T1_4_5/2
  demux16_/7(Out7) -> T1_4_6/2
  demux16_/8(Out8) -> T1_4_7/2
  demux16_/9(Out9) -> T1_4_9/2
  demux16_/10(Out10) -> T1_4_10/2
  demux16_/11(Out11) -> T1_4_11/2
  demux16_/12(Out12) -> T1_4_15/2
  demux16_/13(Out13) -> T1_4_8/2
  demux16_/14(Out14) -> T1_4_12/2
  demux16_/15(Out15) -> T1_4_13/2
  demux16_/16(Out16) -> T1_4_14/2
  T1_4_/1 -> Mux1/2, Mux/2
  T1_4_1/1 -> Mux1/3, Mux/3
  T1_4_2/1 -> Mux1/4, Mux/4
  T1_4_3/1 -> Mux1/5, Mux/5
  T1_4_4/1 -> Mux/6, Mux1/6
  T1_4_5/1 -> Mux1/7, Mux/7
  T1_4_6/1 -> Mux1/8, Mux/8
  T1_4_7/1 -> Mux1/9, Mux/9
  T1_4_9/1 -> Mux1/10, Mux/10
  T1_4_10/1 -> Mux1/11, Mux/11
  T1_4_11/1 -> Mux1/12, Mux/12
  T1_4_15/1 -> Mux1/13, Mux/13
  T1_4_8/1 -> Mux1/14, Mux/14
  T1_4_12/1 -> Mux1/15, Mux/15
  T1_4_13/1 -> Mux1/16, Mux/16
  T1_4_14/1 -> Mux/17, Mux1/17
  Mux/1 -> Out1/1
  chan2/1 -> Mux1/1
  Mux1/1 -> Out2/1

== system fftanalyzeri/FIFO64_2/FIFO32_0/FIFO16Cir_1/CounterArray1 ==
  chan : Inport
  inc : Inport  Port=2
  rst : Inport  Port=3
  Mux : xbsIndex_r4/Mux  inputs=16  en=off  latency=0  precision=Full  arith_type=Unsigned  n_bits=16  bin_pt=14  quantization=Truncate  overflow=Wrap  dbl_ovrd=off  block_type=mux
  T1_4_{,1..15} (16 alike) : xbsIndex_r4/Counter  cnt_type=Free Running  cnt_to=Inf  operation=Up  start_count=0  cnt_by_val=1  arith_type=Unsigned  n_bits=8  bin_pt=0  load_pin=off  rst=on  en=on  explicit_period=on  period=1  dbl_ovrd=off  use_behavioral_HDL=off  implementation=Fabric  block_type=counter
  demux16_ : Subsystem
  Out1 : Outport
  wires:
  chan/1 -> Mux/1, demux16_/1(Chan)
  inc/1 -> demux16_/2(din)
  rst/1 -> T1_4_9/1, T1_4_10/1, T1_4_11/1, T1_4_12/1, T1_4_8/1, T1_4_13/1, T1_4_15/1, T1_4_14/1, T1_4_7/1, T1_4_6/1, T1_4_5/1, T1_4_4/1, T1_4_3/1, T1_4_2/1, T1_4_1/1, T1_4_/1
  demux16_/1(Out1) -> T1_4_/2
  demux16_/2(Out2) -> T1_4_1/2
  demux16_/3(Out3) -> T1_4_2/2
  demux16_/4(Out4) -> T1_4_3/2
  demux16_/5(Out5) -> T1_4_4/2
  demux16_/6(Out6) -> T1_4_5/2
  demux16_/7(Out7) -> T1_4_6/2
  demux16_/8(Out8) -> T1_4_7/2
  demux16_/9(Out9) -> T1_4_9/2
  demux16_/10(Out10) -> T1_4_10/2
  demux16_/11(Out11) -> T1_4_11/2
  demux16_/12(Out12) -> T1_4_12/2
  demux16_/13(Out13) -> T1_4_8/2
  demux16_/14(Out14) -> T1_4_13/2
  demux16_/15(Out15) -> T1_4_14/2
  demux16_/16(Out16) -> T1_4_15/2
  T1_4_/1 -> Mux/2
  T1_4_1/1 -> Mux/3
  T1_4_2/1 -> Mux/4
  T1_4_3/1 -> Mux/5
  T1_4_4/1 -> Mux/6
  T1_4_5/1 -> Mux/7
  T1_4_6/1 -> Mux/8
  T1_4_7/1 -> Mux/9
  T1_4_9/1 -> Mux/10
  T1_4_10/1 -> Mux/11
  T1_4_11/1 -> Mux/12
  T1_4_12/1 -> Mux/13
  T1_4_8/1 -> Mux/14
  T1_4_13/1 -> Mux/15
  T1_4_14/1 -> Mux/16
  T1_4_15/1 -> Mux/17
  Mux/1 -> Out1/1

== system fftanalyzeri/FIFO64_2/FIFO32_0/FIFO16Cir_1/CounterArray2 ==
  chan : Inport
  inc : Inport  Port=2
  rst : Inport  Port=3
  chan2 : Inport  Port=4
  Mux : xbsIndex_r4/Mux  inputs=16  en=off  latency=0  precision=Full  arith_type=Unsigned  n_bits=16  bin_pt=14  quantization=Truncate  overflow=Wrap  dbl_ovrd=off  block_type=mux
  Mux1 : xbsIndex_r4/Mux  inputs=16  en=off  latency=0  precision=Full  arith_type=Unsigned  n_bits=16  bin_pt=14  quantization=Truncate  overflow=Wrap  dbl_ovrd=off  block_type=mux
  T1_4_{,1..15} (16 alike) : xbsIndex_r4/Counter  cnt_type=Free Running  cnt_to=Inf  operation=Up  start_count=0  cnt_by_val=1  arith_type=Unsigned  n_bits=8  bin_pt=0  load_pin=off  rst=on  en=on  explicit_period=on  period=1  dbl_ovrd=off  use_behavioral_HDL=off  implementation=Fabric  block_type=counter
  demux16_ : Subsystem
  Out1 : Outport
  Out2 : Outport  Port=2
  wires:
  chan/1 -> Mux/1, demux16_/1(Chan)
  inc/1 -> demux16_/2(din)
  rst/1 -> T1_4_9/1, T1_4_10/1, T1_4_11/1, T1_4_15/1, T1_4_8/1, T1_4_12/1, T1_4_14/1, T1_4_13/1, T1_4_7/1, T1_4_5/1, T1_4_1/1, T1_4_/1, T1_4_2/1, T1_4_3/1, T1_4_4/1, T1_4_6/1
  demux16_/1(Out1) -> T1_4_/2
  demux16_/2(Out2) -> T1_4_1/2
  demux16_/3(Out3) -> T1_4_2/2
  demux16_/4(Out4) -> T1_4_3/2
  demux16_/5(Out5) -> T1_4_4/2
  demux16_/6(Out6) -> T1_4_5/2
  demux16_/7(Out7) -> T1_4_6/2
  demux16_/8(Out8) -> T1_4_7/2
  demux16_/9(Out9) -> T1_4_9/2
  demux16_/10(Out10) -> T1_4_10/2
  demux16_/11(Out11) -> T1_4_11/2
  demux16_/12(Out12) -> T1_4_15/2
  demux16_/13(Out13) -> T1_4_8/2
  demux16_/14(Out14) -> T1_4_12/2
  demux16_/15(Out15) -> T1_4_13/2
  demux16_/16(Out16) -> T1_4_14/2
  T1_4_/1 -> Mux1/2, Mux/2
  T1_4_1/1 -> Mux1/3, Mux/3
  T1_4_2/1 -> Mux1/4, Mux/4
  T1_4_3/1 -> Mux1/5, Mux/5
  T1_4_4/1 -> Mux/6, Mux1/6
  T1_4_5/1 -> Mux1/7, Mux/7
  T1_4_6/1 -> Mux1/8, Mux/8
  T1_4_7/1 -> Mux1/9, Mux/9
  T1_4_9/1 -> Mux1/10, Mux/10
  T1_4_10/1 -> Mux1/11, Mux/11
  T1_4_11/1 -> Mux1/12, Mux/12
  T1_4_15/1 -> Mux1/13, Mux/13
  T1_4_8/1 -> Mux1/14, Mux/14
  T1_4_12/1 -> Mux1/15, Mux/15
  T1_4_13/1 -> Mux1/16, Mux/16
  T1_4_14/1 -> Mux/17, Mux1/17
  Mux/1 -> Out1/1
  chan2/1 -> Mux1/1
  Mux1/1 -> Out2/1

== system fftanalyzeri/FIFO64_2/FIFO32_0/FIFO16Cir_2/CounterArray1 ==
  chan : Inport
  inc : Inport  Port=2
  rst : Inport  Port=3
  Mux : xbsIndex_r4/Mux  inputs=16  en=off  latency=0  precision=Full  arith_type=Unsigned  n_bits=16  bin_pt=14  quantization=Truncate  overflow=Wrap  dbl_ovrd=off  block_type=mux
  T1_4_{,1..15} (16 alike) : xbsIndex_r4/Counter  cnt_type=Free Running  cnt_to=Inf  operation=Up  start_count=0  cnt_by_val=1  arith_type=Unsigned  n_bits=8  bin_pt=0  load_pin=off  rst=on  en=on  explicit_period=on  period=1  dbl_ovrd=off  use_behavioral_HDL=off  implementation=Fabric  block_type=counter
  demux16_ : Subsystem
  Out1 : Outport
  wires:
  chan/1 -> Mux/1, demux16_/1(Chan)
  inc/1 -> demux16_/2(din)
  rst/1 -> T1_4_9/1, T1_4_10/1, T1_4_11/1, T1_4_12/1, T1_4_8/1, T1_4_13/1, T1_4_15/1, T1_4_14/1, T1_4_7/1, T1_4_6/1, T1_4_5/1, T1_4_4/1, T1_4_3/1, T1_4_2/1, T1_4_1/1, T1_4_/1
  demux16_/1(Out1) -> T1_4_/2
  demux16_/2(Out2) -> T1_4_1/2
  demux16_/3(Out3) -> T1_4_2/2
  demux16_/4(Out4) -> T1_4_3/2
  demux16_/5(Out5) -> T1_4_4/2
  demux16_/6(Out6) -> T1_4_5/2
  demux16_/7(Out7) -> T1_4_6/2
  demux16_/8(Out8) -> T1_4_7/2
  demux16_/9(Out9) -> T1_4_9/2
  demux16_/10(Out10) -> T1_4_10/2
  demux16_/11(Out11) -> T1_4_11/2
  demux16_/12(Out12) -> T1_4_12/2
  demux16_/13(Out13) -> T1_4_8/2
  demux16_/14(Out14) -> T1_4_13/2
  demux16_/15(Out15) -> T1_4_14/2
  demux16_/16(Out16) -> T1_4_15/2
  T1_4_/1 -> Mux/2
  T1_4_1/1 -> Mux/3
  T1_4_2/1 -> Mux/4
  T1_4_3/1 -> Mux/5
  T1_4_4/1 -> Mux/6
  T1_4_5/1 -> Mux/7
  T1_4_6/1 -> Mux/8
  T1_4_7/1 -> Mux/9
  T1_4_9/1 -> Mux/10
  T1_4_10/1 -> Mux/11
  T1_4_11/1 -> Mux/12
  T1_4_12/1 -> Mux/13
  T1_4_8/1 -> Mux/14
  T1_4_13/1 -> Mux/15
  T1_4_14/1 -> Mux/16
  T1_4_15/1 -> Mux/17
  Mux/1 -> Out1/1

== system fftanalyzeri/FIFO64_2/FIFO32_0/FIFO16Cir_2/CounterArray2 ==
  chan : Inport
  inc : Inport  Port=2
  rst : Inport  Port=3
  chan2 : Inport  Port=4
  Mux : xbsIndex_r4/Mux  inputs=16  en=off  latency=0  precision=Full  arith_type=Unsigned  n_bits=16  bin_pt=14  quantization=Truncate  overflow=Wrap  dbl_ovrd=off  block_type=mux
  Mux1 : xbsIndex_r4/Mux  inputs=16  en=off  latency=0  precision=Full  arith_type=Unsigned  n_bits=16  bin_pt=14  quantization=Truncate  overflow=Wrap  dbl_ovrd=off  block_type=mux
  T1_4_{,1..15} (16 alike) : xbsIndex_r4/Counter  cnt_type=Free Running  cnt_to=Inf  operation=Up  start_count=0  cnt_by_val=1  arith_type=Unsigned  n_bits=8  bin_pt=0  load_pin=off  rst=on  en=on  explicit_period=on  period=1  dbl_ovrd=off  use_behavioral_HDL=off  implementation=Fabric  block_type=counter
  demux16_ : Subsystem
  Out1 : Outport
  Out2 : Outport  Port=2
  wires:
  chan/1 -> Mux/1, demux16_/1(Chan)
  inc/1 -> demux16_/2(din)
  rst/1 -> T1_4_9/1, T1_4_10/1, T1_4_11/1, T1_4_15/1, T1_4_8/1, T1_4_12/1, T1_4_14/1, T1_4_13/1, T1_4_7/1, T1_4_5/1, T1_4_1/1, T1_4_/1, T1_4_2/1, T1_4_3/1, T1_4_4/1, T1_4_6/1
  demux16_/1(Out1) -> T1_4_/2
  demux16_/2(Out2) -> T1_4_1/2
  demux16_/3(Out3) -> T1_4_2/2
  demux16_/4(Out4) -> T1_4_3/2
  demux16_/5(Out5) -> T1_4_4/2
  demux16_/6(Out6) -> T1_4_5/2
  demux16_/7(Out7) -> T1_4_6/2
  demux16_/8(Out8) -> T1_4_7/2
  demux16_/9(Out9) -> T1_4_9/2
  demux16_/10(Out10) -> T1_4_10/2
  demux16_/11(Out11) -> T1_4_11/2
  demux16_/12(Out12) -> T1_4_15/2
  demux16_/13(Out13) -> T1_4_8/2
  demux16_/14(Out14) -> T1_4_12/2
  demux16_/15(Out15) -> T1_4_13/2
  demux16_/16(Out16) -> T1_4_14/2
  T1_4_/1 -> Mux1/2, Mux/2
  T1_4_1/1 -> Mux1/3, Mux/3
  T1_4_2/1 -> Mux1/4, Mux/4
  T1_4_3/1 -> Mux1/5, Mux/5
  T1_4_4/1 -> Mux/6, Mux1/6
  T1_4_5/1 -> Mux1/7, Mux/7
  T1_4_6/1 -> Mux1/8, Mux/8
  T1_4_7/1 -> Mux1/9, Mux/9
  T1_4_9/1 -> Mux1/10, Mux/10
  T1_4_10/1 -> Mux1/11, Mux/11
  T1_4_11/1 -> Mux1/12, Mux/12
  T1_4_15/1 -> Mux1/13, Mux/13
  T1_4_8/1 -> Mux1/14, Mux/14
  T1_4_12/1 -> Mux1/15, Mux/15
  T1_4_13/1 -> Mux1/16, Mux/16
  T1_4_14/1 -> Mux/17, Mux1/17
  Mux/1 -> Out1/1
  chan2/1 -> Mux1/1
  Mux1/1 -> Out2/1

== system fftanalyzeri/FIFO64_2/FIFO32_1/FIFO16Cir_1/CounterArray1 ==
  chan : Inport
  inc : Inport  Port=2
  rst : Inport  Port=3
  Mux : xbsIndex_r4/Mux  inputs=16  en=off  latency=0  precision=Full  arith_type=Unsigned  n_bits=16  bin_pt=14  quantization=Truncate  overflow=Wrap  dbl_ovrd=off  block_type=mux
  T1_4_{,1..15} (16 alike) : xbsIndex_r4/Counter  cnt_type=Free Running  cnt_to=Inf  operation=Up  start_count=0  cnt_by_val=1  arith_type=Unsigned  n_bits=8  bin_pt=0  load_pin=off  rst=on  en=on  explicit_period=on  period=1  dbl_ovrd=off  use_behavioral_HDL=off  implementation=Fabric  block_type=counter
  demux16_ : Subsystem
  Out1 : Outport
  wires:
  chan/1 -> Mux/1, demux16_/1(Chan)
  inc/1 -> demux16_/2(din)
  rst/1 -> T1_4_9/1, T1_4_10/1, T1_4_11/1, T1_4_12/1, T1_4_8/1, T1_4_13/1, T1_4_15/1, T1_4_14/1, T1_4_7/1, T1_4_6/1, T1_4_5/1, T1_4_4/1, T1_4_3/1, T1_4_2/1, T1_4_1/1, T1_4_/1
  demux16_/1(Out1) -> T1_4_/2
  demux16_/2(Out2) -> T1_4_1/2
  demux16_/3(Out3) -> T1_4_2/2
  demux16_/4(Out4) -> T1_4_3/2
  demux16_/5(Out5) -> T1_4_4/2
  demux16_/6(Out6) -> T1_4_5/2
  demux16_/7(Out7) -> T1_4_6/2
  demux16_/8(Out8) -> T1_4_7/2
  demux16_/9(Out9) -> T1_4_9/2
  demux16_/10(Out10) -> T1_4_10/2
  demux16_/11(Out11) -> T1_4_11/2
  demux16_/12(Out12) -> T1_4_12/2
  demux16_/13(Out13) -> T1_4_8/2
  demux16_/14(Out14) -> T1_4_13/2
  demux16_/15(Out15) -> T1_4_14/2
  demux16_/16(Out16) -> T1_4_15/2
  T1_4_/1 -> Mux/2
  T1_4_1/1 -> Mux/3
  T1_4_2/1 -> Mux/4
  T1_4_3/1 -> Mux/5
  T1_4_4/1 -> Mux/6
  T1_4_5/1 -> Mux/7
  T1_4_6/1 -> Mux/8
  T1_4_7/1 -> Mux/9
  T1_4_9/1 -> Mux/10
  T1_4_10/1 -> Mux/11
  T1_4_11/1 -> Mux/12
  T1_4_12/1 -> Mux/13
  T1_4_8/1 -> Mux/14
  T1_4_13/1 -> Mux/15
  T1_4_14/1 -> Mux/16
  T1_4_15/1 -> Mux/17
  Mux/1 -> Out1/1

== system fftanalyzeri/FIFO64_2/FIFO32_1/FIFO16Cir_1/CounterArray2 ==
  chan : Inport
  inc : Inport  Port=2
  rst : Inport  Port=3
  chan2 : Inport  Port=4
  Mux : xbsIndex_r4/Mux  inputs=16  en=off  latency=0  precision=Full  arith_type=Unsigned  n_bits=16  bin_pt=14  quantization=Truncate  overflow=Wrap  dbl_ovrd=off  block_type=mux
  Mux1 : xbsIndex_r4/Mux  inputs=16  en=off  latency=0  precision=Full  arith_type=Unsigned  n_bits=16  bin_pt=14  quantization=Truncate  overflow=Wrap  dbl_ovrd=off  block_type=mux
  T1_4_{,1..15} (16 alike) : xbsIndex_r4/Counter  cnt_type=Free Running  cnt_to=Inf  operation=Up  start_count=0  cnt_by_val=1  arith_type=Unsigned  n_bits=8  bin_pt=0  load_pin=off  rst=on  en=on  explicit_period=on  period=1  dbl_ovrd=off  use_behavioral_HDL=off  implementation=Fabric  block_type=counter
  demux16_ : Subsystem
  Out1 : Outport
  Out2 : Outport  Port=2
  wires:
  chan/1 -> Mux/1, demux16_/1(Chan)
  inc/1 -> demux16_/2(din)
  rst/1 -> T1_4_9/1, T1_4_10/1, T1_4_11/1, T1_4_15/1, T1_4_8/1, T1_4_12/1, T1_4_14/1, T1_4_13/1, T1_4_7/1, T1_4_5/1, T1_4_1/1, T1_4_/1, T1_4_2/1, T1_4_3/1, T1_4_4/1, T1_4_6/1
  demux16_/1(Out1) -> T1_4_/2
  demux16_/2(Out2) -> T1_4_1/2
  demux16_/3(Out3) -> T1_4_2/2
  demux16_/4(Out4) -> T1_4_3/2
  demux16_/5(Out5) -> T1_4_4/2
  demux16_/6(Out6) -> T1_4_5/2
  demux16_/7(Out7) -> T1_4_6/2
  demux16_/8(Out8) -> T1_4_7/2
  demux16_/9(Out9) -> T1_4_9/2
  demux16_/10(Out10) -> T1_4_10/2
  demux16_/11(Out11) -> T1_4_11/2
  demux16_/12(Out12) -> T1_4_15/2
  demux16_/13(Out13) -> T1_4_8/2
  demux16_/14(Out14) -> T1_4_12/2
  demux16_/15(Out15) -> T1_4_13/2
  demux16_/16(Out16) -> T1_4_14/2
  T1_4_/1 -> Mux1/2, Mux/2
  T1_4_1/1 -> Mux1/3, Mux/3
  T1_4_2/1 -> Mux1/4, Mux/4
  T1_4_3/1 -> Mux1/5, Mux/5
  T1_4_4/1 -> Mux/6, Mux1/6
  T1_4_5/1 -> Mux1/7, Mux/7
  T1_4_6/1 -> Mux1/8, Mux/8
  T1_4_7/1 -> Mux1/9, Mux/9
  T1_4_9/1 -> Mux1/10, Mux/10
  T1_4_10/1 -> Mux1/11, Mux/11
  T1_4_11/1 -> Mux1/12, Mux/12
  T1_4_15/1 -> Mux1/13, Mux/13
  T1_4_8/1 -> Mux1/14, Mux/14
  T1_4_12/1 -> Mux1/15, Mux/15
  T1_4_13/1 -> Mux1/16, Mux/16
  T1_4_14/1 -> Mux/17, Mux1/17
  Mux/1 -> Out1/1
  chan2/1 -> Mux1/1
  Mux1/1 -> Out2/1

== system fftanalyzeri/FIFO64_2/FIFO32_1/FIFO16Cir_2/CounterArray1 ==
  chan : Inport
  inc : Inport  Port=2
  rst : Inport  Port=3
  Mux : xbsIndex_r4/Mux  inputs=16  en=off  latency=0  precision=Full  arith_type=Unsigned  n_bits=16  bin_pt=14  quantization=Truncate  overflow=Wrap  dbl_ovrd=off  block_type=mux
  T1_4_{,1..15} (16 alike) : xbsIndex_r4/Counter  cnt_type=Free Running  cnt_to=Inf  operation=Up  start_count=0  cnt_by_val=1  arith_type=Unsigned  n_bits=8  bin_pt=0  load_pin=off  rst=on  en=on  explicit_period=on  period=1  dbl_ovrd=off  use_behavioral_HDL=off  implementation=Fabric  block_type=counter
  demux16_ : Subsystem
  Out1 : Outport
  wires:
  chan/1 -> Mux/1, demux16_/1(Chan)
  inc/1 -> demux16_/2(din)
  rst/1 -> T1_4_9/1, T1_4_10/1, T1_4_11/1, T1_4_12/1, T1_4_8/1, T1_4_13/1, T1_4_15/1, T1_4_14/1, T1_4_7/1, T1_4_6/1, T1_4_5/1, T1_4_4/1, T1_4_3/1, T1_4_2/1, T1_4_1/1, T1_4_/1
  demux16_/1(Out1) -> T1_4_/2
  demux16_/2(Out2) -> T1_4_1/2
  demux16_/3(Out3) -> T1_4_2/2
  demux16_/4(Out4) -> T1_4_3/2
  demux16_/5(Out5) -> T1_4_4/2
  demux16_/6(Out6) -> T1_4_5/2
  demux16_/7(Out7) -> T1_4_6/2
  demux16_/8(Out8) -> T1_4_7/2
  demux16_/9(Out9) -> T1_4_9/2
  demux16_/10(Out10) -> T1_4_10/2
  demux16_/11(Out11) -> T1_4_11/2
  demux16_/12(Out12) -> T1_4_12/2
  demux16_/13(Out13) -> T1_4_8/2
  demux16_/14(Out14) -> T1_4_13/2
  demux16_/15(Out15) -> T1_4_14/2
  demux16_/16(Out16) -> T1_4_15/2
  T1_4_/1 -> Mux/2
  T1_4_1/1 -> Mux/3
  T1_4_2/1 -> Mux/4
  T1_4_3/1 -> Mux/5
  T1_4_4/1 -> Mux/6
  T1_4_5/1 -> Mux/7
  T1_4_6/1 -> Mux/8
  T1_4_7/1 -> Mux/9
  T1_4_9/1 -> Mux/10
  T1_4_10/1 -> Mux/11
  T1_4_11/1 -> Mux/12
  T1_4_12/1 -> Mux/13
  T1_4_8/1 -> Mux/14
  T1_4_13/1 -> Mux/15
  T1_4_14/1 -> Mux/16
  T1_4_15/1 -> Mux/17
  Mux/1 -> Out1/1

== system fftanalyzeri/FIFO64_2/FIFO32_1/FIFO16Cir_2/CounterArray2 ==
  chan : Inport
  inc : Inport  Port=2
  rst : Inport  Port=3
  chan2 : Inport  Port=4
  Mux : xbsIndex_r4/Mux  inputs=16  en=off  latency=0  precision=Full  arith_type=Unsigned  n_bits=16  bin_pt=14  quantization=Truncate  overflow=Wrap  dbl_ovrd=off  block_type=mux
  Mux1 : xbsIndex_r4/Mux  inputs=16  en=off  latency=0  precision=Full  arith_type=Unsigned  n_bits=16  bin_pt=14  quantization=Truncate  overflow=Wrap  dbl_ovrd=off  block_type=mux
  T1_4_{,1..15} (16 alike) : xbsIndex_r4/Counter  cnt_type=Free Running  cnt_to=Inf  operation=Up  start_count=0  cnt_by_val=1  arith_type=Unsigned  n_bits=8  bin_pt=0  load_pin=off  rst=on  en=on  explicit_period=on  period=1  dbl_ovrd=off  use_behavioral_HDL=off  implementation=Fabric  block_type=counter
  demux16_ : Subsystem
  Out1 : Outport
  Out2 : Outport  Port=2
  wires:
  chan/1 -> Mux/1, demux16_/1(Chan)
  inc/1 -> demux16_/2(din)
  rst/1 -> T1_4_9/1, T1_4_10/1, T1_4_11/1, T1_4_15/1, T1_4_8/1, T1_4_12/1, T1_4_14/1, T1_4_13/1, T1_4_7/1, T1_4_5/1, T1_4_1/1, T1_4_/1, T1_4_2/1, T1_4_3/1, T1_4_4/1, T1_4_6/1
  demux16_/1(Out1) -> T1_4_/2
  demux16_/2(Out2) -> T1_4_1/2
  demux16_/3(Out3) -> T1_4_2/2
  demux16_/4(Out4) -> T1_4_3/2
  demux16_/5(Out5) -> T1_4_4/2
  demux16_/6(Out6) -> T1_4_5/2
  demux16_/7(Out7) -> T1_4_6/2
  demux16_/8(Out8) -> T1_4_7/2
  demux16_/9(Out9) -> T1_4_9/2
  demux16_/10(Out10) -> T1_4_10/2
  demux16_/11(Out11) -> T1_4_11/2
  demux16_/12(Out12) -> T1_4_15/2
  demux16_/13(Out13) -> T1_4_8/2
  demux16_/14(Out14) -> T1_4_12/2
  demux16_/15(Out15) -> T1_4_13/2
  demux16_/16(Out16) -> T1_4_14/2
  T1_4_/1 -> Mux1/2, Mux/2
  T1_4_1/1 -> Mux1/3, Mux/3
  T1_4_2/1 -> Mux1/4, Mux/4
  T1_4_3/1 -> Mux1/5, Mux/5
  T1_4_4/1 -> Mux/6, Mux1/6
  T1_4_5/1 -> Mux1/7, Mux/7
  T1_4_6/1 -> Mux1/8, Mux/8
  T1_4_7/1 -> Mux1/9, Mux/9
  T1_4_9/1 -> Mux1/10, Mux/10
  T1_4_10/1 -> Mux1/11, Mux/11
  T1_4_11/1 -> Mux1/12, Mux/12
  T1_4_15/1 -> Mux1/13, Mux/13
  T1_4_8/1 -> Mux1/14, Mux/14
  T1_4_12/1 -> Mux1/15, Mux/15
  T1_4_13/1 -> Mux1/16, Mux/16
  T1_4_14/1 -> Mux/17, Mux1/17
  Mux/1 -> Out1/1
  chan2/1 -> Mux1/1
  Mux1/1 -> Out2/1

== system fftanalyzeri/FIFO64_3/FIFO32_0/FIFO16Cir_1/CounterArray1 ==
  chan : Inport
  inc : Inport  Port=2
  rst : Inport  Port=3
  Mux : xbsIndex_r4/Mux  inputs=16  en=off  latency=0  precision=Full  arith_type=Unsigned  n_bits=16  bin_pt=14  quantization=Truncate  overflow=Wrap  dbl_ovrd=off  block_type=mux
  T1_4_{,1..15} (16 alike) : xbsIndex_r4/Counter  cnt_type=Free Running  cnt_to=Inf  operation=Up  start_count=0  cnt_by_val=1  arith_type=Unsigned  n_bits=8  bin_pt=0  load_pin=off  rst=on  en=on  explicit_period=on  period=1  dbl_ovrd=off  use_behavioral_HDL=off  implementation=Fabric  block_type=counter
  demux16_ : Subsystem
  Out1 : Outport
  wires:
  chan/1 -> Mux/1, demux16_/1(Chan)
  inc/1 -> demux16_/2(din)
  rst/1 -> T1_4_9/1, T1_4_10/1, T1_4_11/1, T1_4_12/1, T1_4_8/1, T1_4_13/1, T1_4_15/1, T1_4_14/1, T1_4_7/1, T1_4_6/1, T1_4_5/1, T1_4_4/1, T1_4_3/1, T1_4_2/1, T1_4_1/1, T1_4_/1
  demux16_/1(Out1) -> T1_4_/2
  demux16_/2(Out2) -> T1_4_1/2
  demux16_/3(Out3) -> T1_4_2/2
  demux16_/4(Out4) -> T1_4_3/2
  demux16_/5(Out5) -> T1_4_4/2
  demux16_/6(Out6) -> T1_4_5/2
  demux16_/7(Out7) -> T1_4_6/2
  demux16_/8(Out8) -> T1_4_7/2
  demux16_/9(Out9) -> T1_4_9/2
  demux16_/10(Out10) -> T1_4_10/2
  demux16_/11(Out11) -> T1_4_11/2
  demux16_/12(Out12) -> T1_4_12/2
  demux16_/13(Out13) -> T1_4_8/2
  demux16_/14(Out14) -> T1_4_13/2
  demux16_/15(Out15) -> T1_4_14/2
  demux16_/16(Out16) -> T1_4_15/2
  T1_4_/1 -> Mux/2
  T1_4_1/1 -> Mux/3
  T1_4_2/1 -> Mux/4
  T1_4_3/1 -> Mux/5
  T1_4_4/1 -> Mux/6
  T1_4_5/1 -> Mux/7
  T1_4_6/1 -> Mux/8
  T1_4_7/1 -> Mux/9
  T1_4_9/1 -> Mux/10
  T1_4_10/1 -> Mux/11
  T1_4_11/1 -> Mux/12
  T1_4_12/1 -> Mux/13
  T1_4_8/1 -> Mux/14
  T1_4_13/1 -> Mux/15
  T1_4_14/1 -> Mux/16
  T1_4_15/1 -> Mux/17
  Mux/1 -> Out1/1
